simulink model "MoveMove"  (R2018a)
settings: Solver=ode4  StartTime=0.0  StopTime=19  FixedStep=5e-4  RelTol=1e-2
PostLoadFcn:
  | helperSetUp
values from neighbouring files (symbols this model uses):
  bf = 12    [data_vehicle.m]    (also in matlab.mat; testMotionPlanner.mat)
  br = 14    [data_vehicle.m]    (also in matlab.mat; testMotionPlanner.mat)
  Cd = .3    (= 0.3)    [data_vehicle.m]    (also in matlab.mat; myVehicle.m = this.CD; testMotionPlanner.mat)
  Cf = 1.3    [data_vehicle.m]    (also in forwardPropagate.m = 19000; matlab.mat; myVehicle.m = this.CF; testMotionPlanner.mat)
  costmap = vehicleCostmap(combinedMap, 'CellSize', res)    [creatCostmap.m]    (also in creatMyCostMap.m = vehicleCostmap(combinedMap, 'CellSize', res,                ; myMotionPlanning.m = vehicleCostmap(costmapStruct.Costs,          'FreeThreshold')
  Cr = 1.3    [data_vehicle.m]    (also in forwardPropagate.m = 33000; matlab.mat; myVehicle.m = this.CR; testMotionPlanner.mat)
  df = 0.95    [data_vehicle.m]    (also in matlab.mat; testMotionPlanner.mat)
  dr = 1    [data_vehicle.m]    (also in matlab.mat; testMotionPlanner.mat)
  Ef = -0.1    [data_vehicle.m]    (also in matlab.mat; testMotionPlanner.mat)
  Er = -0.1    [data_vehicle.m]    (also in matlab.mat; testMotionPlanner.mat)
  fv = .02    (= 0.02)    [data_vehicle.m]    (also in matlab.mat; testMotionPlanner.mat)
  Fzf = m*g*lr/l    (= 9879.29185185)    [data_vehicle.m]    (also in matlab.mat; testMotionPlanner.mat)
  Fzr = m*g*lf/l    (= 5811.34814815)    [data_vehicle.m]    (also in matlab.mat; testMotionPlanner.mat)
  g = 9.80665    [data_vehicle.m]    (also in matlab.mat; myVehicle.m = this.G; testMotionPlanner.mat)
  gB = 2/3    (= 0.666666666667)    [data_vehicle.m]    (also in matlab.mat; testMotionPlanner.mat)
  gT = 0    [data_vehicle.m]    (also in matlab.mat; testMotionPlanner.mat)
  Jz = 2200    [data_vehicle.m]    (also in matlab.mat; testMotionPlanner.mat)
  lf = 1    [data_vehicle.m]    (also in forwardPropagate.m = 1.2; matlab.mat; myVehicle.m = this.LF; testMotionPlanner.mat)
  lr = l-lf    (= 1.7)    [data_vehicle.m]    (also in forwardPropagate.m = 1.6; matlab.mat; myVehicle.m = this.LR; testMotionPlanner.mat)
  m = 1600    [data_vehicle.m]    (also in forwardPropagate.m = 1575; matlab.mat; myVehicle.m = this.M; testMotionPlanner.mat)
  mu = 1    [data_vehicle.m]    (also in matlab.mat; myVehicle.m = this.MU; testMotionPlanner.mat)
  psi0 = 0    [data_vehicle.m]    (also in matlab.mat; testMotionPlanner.mat)
  psip0 = 0    [data_vehicle.m]    (also in matlab.mat; testMotionPlanner.mat)
  rho = 1.2    [data_vehicle.m]    (also in matlab.mat; myVehicle.m = 1.29; testMotionPlanner.mat)
  S = 2    [data_vehicle.m]    (also in matlab.mat; testMotionPlanner.mat)
  vx0 = 0    [data_vehicle.m]    (also in matlab.mat; testMotionPlanner.mat)
  vy0 = 0    [data_vehicle.m]    (also in matlab.mat; testMotionPlanner.mat)
  XG0 = 0    [data_vehicle.m]    (also in matlab.mat; testMotionPlanner.mat)
  YG0 = 0    [data_vehicle.m]    (also in matlab.mat; testMotionPlanner.mat)
undefined symbols (not defined in the file or in its folder): dt_save
settings Model: Creator=jdrjk  LastModifiedBy=jdrjk

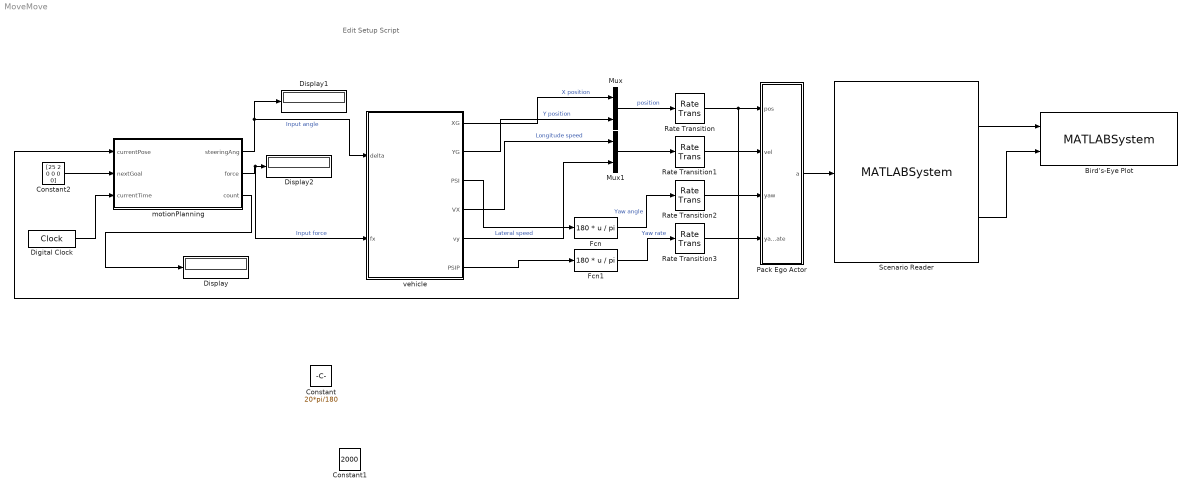
== system MoveMove ==
  note: Edit Setup Script
  Bird's-Eye Plot : MATLABSystem  System=helperBirdsEyePlot  ScenarioFileName=lkaScenarioSimulink  XLim=[-20, 50 ]  YLim=[ -30, 30 ]  HasActors=on  HasVision=off  HasRadar=off  HasTracks=off  TrackPositionSelector=[ 1, 0, 0, 0, 0, 0; 0, 0, 1, 0, 0, 0 ]  TrackVelocitySelector=[ 0, 1, 0, 0, 0, 0; 0, 0, 0, 1, 0, 0 ]  HasMIO=off  HasRoads=off  HasLaneBoundaries=off  HasLaneMarkings=on
      settings: ModelCloseFcn=helperCloseAll(gcb)
      mask Type: helperBirdsEyePlot
      mask Display:
      | disp(['Bird''s-Eye' char(10) 'Plot']);
      | port_label('input',1,'Actors');
      | port_label('input',2,'Lane Markings');
  Constant : Constant  Value=20*pi/180
  Constant1 : Constant  Value=2000
  Constant2 : Constant  Value=[25 2 0 0 0 0]  VectorParams1D=off
  Digital Clock : DigitalClock  SampleTime=0.01
  Display : Display
  Display1 : Display
  Display2 : Display
  Fcn : Fcn  Expr=180 * u / pi
  Fcn1 : Fcn  Expr=180 * u / pi
  Mux : Mux  Inputs=2
  Mux1 : Mux  Inputs=2
  Pack Ego Actor : MATLAB Function  TreatAsAtomicUnit=on
  Rate Transition{,1..3} (4 alike) : RateTransition  OutPortSampleTime=Ts
  Scenario Reader : MATLABSystem  System=helperScenarioReader  ScenarioFileName=lkaScenarioSimulink  EgoActorSource=Input port  EgoActorID=1  RoadBoundaries=off  LaneBoundaries=off  AllBoundaries=off  LaneBoundaryDistance=0:0.5:60  LaneBoundaryLocation=inner  CurrentLane=off  NumLanes=off  LaneMarkings=on  BusNameSource=Auto  BusName2Source=Auto  BusName3Source=Auto  SimulateUsing=Interpreted execution
      mask Type: helperScenarioReader
      mask Display:
      | disp(['Scenario' char(10) 'Reader']);
      | port_label('input',1,'Ego Actor');
      | port_label('output',1,'Actors');
      | port_label('output',2,'Lane Markings');
  motionPlanning : MATLAB Function  TreatAsAtomicUnit=on  mask{Costmap=costmap, MinIterations=1000, ConnectionDistance=3, MinTurningRadius=20, XStart=0, YStart=0, ThetaStart=0}
      mask prompts: Costmap "Vehicle costmap:"; MinIterations "Minimum iteration:"; ConnectionDistance "Connection distance [m]:"; MinTurningRadius "Minimum turning radius [m]:"; XStart "X positon [m]:"; YStart "Y position [m]:"; ThetaStart "Heading angle [deg]:"
      mask init:
      | validateattributes(Costmap, {'vehicleCostmap'}, {'scalar'});
      | 
      | startPose         = [XStart YStart ThetaStart 0 0 0];
      | varagout          = helperSLCreateUtilityStruct(Costmap);
      | vehicleDimsStruct = varagout{1};
      | costmapStruct     = varagout{2};
  vehicle : Subsystem
  wires:
  vehicle/4(VX) -> Mux1/1  "Longitude speed"
  vehicle/2(YG) -> Mux/2  "Y position"
  vehicle/5(vy) -> Mux1/2  "Lateral speed"
  vehicle/3(PSI) -> Fcn/1
  vehicle/1(XG) -> Mux/1  "X position"
  vehicle/6("PSIP ") -> Fcn1/1
  Rate Transition2/1 -> Pack Ego Actor/3(yaw)
  Mux1/1 -> Rate Transition1/1
  Rate Transition/1 -> motionPlanning/1(currentPose), Pack Ego Actor/1(pos)
  Scenario Reader/1 -> Bird's-Eye Plot/1
  Fcn1/1 -> Rate Transition3/1  "Yaw rate"
  Mux/1 -> Rate Transition/1  "position"
  Pack Ego Actor/1(a) -> Scenario Reader/1
  Rate Transition3/1 -> Pack Ego Actor/4(yawRate)
  Rate Transition1/1 -> Pack Ego Actor/2(vel)
  Fcn/1 -> Rate Transition2/1  "Yaw angle"
  Scenario Reader/2 -> Bird's-Eye Plot/2
  Constant2/1 -> motionPlanning/2(nextGoal)
  motionPlanning/2(force) -> vehicle/2(fx), Display2/1  "Input force"
  motionPlanning/3(count) -> Display/1
  Digital Clock/1 -> motionPlanning/3(currentTime)
  motionPlanning/1(steeringAng) -> vehicle/1(delta), Display1/1  "Input angle"

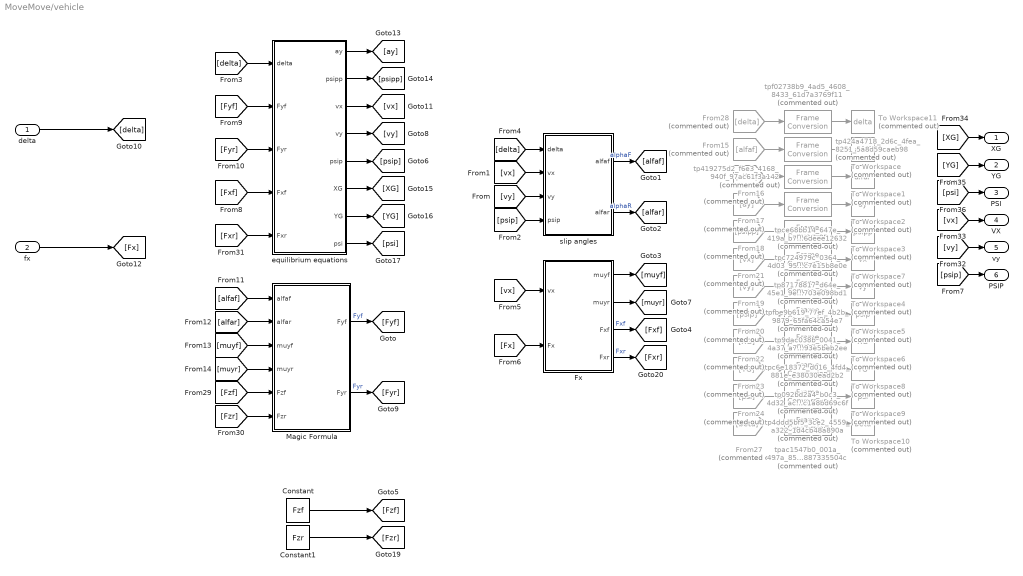
== system MoveMove/vehicle ==
  delta : Inport
  fx : Inport  Port=2
  Constant : Constant  Value=Fzf
  Constant1 : Constant  Value=Fzr
  From15 : From  Commented=on  GotoTag=alfaf
  From16 : From  Commented=on  GotoTag=alfar
  From17 : From  Commented=on  GotoTag=ay
  From18 : From  Commented=on  GotoTag=psipp
  From19 : From  Commented=on  GotoTag=vy
  From20 : From  Commented=on  GotoTag=psip
  From21 : From  Commented=on  GotoTag=vx
  From22 : From  Commented=on  GotoTag=XG
  From23 : From  Commented=on  GotoTag=YG
  From24 : From  Commented=on  GotoTag=psi
  From27 : From  Commented=on  GotoTag=beta
  From28 : From  Commented=on  GotoTag=delta
  Fx : Subsystem
  Magic Formula : Subsystem
  To Workspace : ToWorkspace  Commented=on  VariableName=alfaf  SampleTime=dt_save
  To Workspace1 : ToWorkspace  Commented=on  VariableName=alfar  SampleTime=dt_save
  To Workspace10 : ToWorkspace  Commented=on  VariableName=beta  SampleTime=dt_save
  To Workspace11 : ToWorkspace  Commented=on  VariableName=delta  SampleTime=dt_save
  To Workspace2 : ToWorkspace  Commented=on  VariableName=ay  SampleTime=dt_save
  To Workspace3 : ToWorkspace  Commented=on  VariableName=psipp  SampleTime=dt_save
  To Workspace4 : ToWorkspace  Commented=on  VariableName=vy  SampleTime=dt_save
  To Workspace5 : ToWorkspace  Commented=on  VariableName=psip  SampleTime=dt_save
  To Workspace6 : ToWorkspace  Commented=on  VariableName=XG  SampleTime=dt_save
  To Workspace7 : ToWorkspace  Commented=on  VariableName=vx  SampleTime=dt_save
  To Workspace8 : ToWorkspace  Commented=on  VariableName=YG  SampleTime=dt_save
  To Workspace9 : ToWorkspace  Commented=on  VariableName=psi  SampleTime=dt_save
  equilibrium equations : Subsystem
  slip angles : Subsystem
  tp092bd2a4_b0c3_4d32_ac59_7c1a8bd69c6f : FrameConversion  Commented=on  OutFrame=Sample-based
  tp419275d2_f6e3_4168_940f_97ac61f3a142 : FrameConversion  Commented=on  OutFrame=Sample-based
  tp424a4718_2d6c_4fea_8251_5a8d59caeb98 : FrameConversion  Commented=on  OutFrame=Sample-based
  tp4ddd5bf5_3ce2_4559_a322_1d4cb48a890a : FrameConversion  Commented=on  OutFrame=Sample-based
  tp87178817_d64e_45e1_9e30_db703e098bd1 : FrameConversion  Commented=on  OutFrame=Sample-based
  tp9dac038b_0041_4a37_a752_0593e5beb2ee : FrameConversion  Commented=on  OutFrame=Sample-based
  tpac1547b0_001a_497a_857c_68887335504c : FrameConversion  Commented=on  OutFrame=Sample-based
  tpc6e18372_d016_4fd4_881e_e38030ead2b2 : FrameConversion  Commented=on  OutFrame=Sample-based
  tpc724979c_0364_4d03_952a_37c7e15b8e0e : FrameConversion  Commented=on  OutFrame=Sample-based
  tpce68bb14_647e_419a_b744_5f6deee12632 : FrameConversion  Commented=on  OutFrame=Sample-based
  tpf02738b9_4ad5_4608_8433_61d7a3769f11 : FrameConversion  Commented=on  OutFrame=Sample-based
  tpfbe9b619_77ef_4b2b_9879_65fa64ca54e7 : FrameConversion  Commented=on  OutFrame=Sample-based
  XG : Outport
  YG : Outport  Port=2
  PSI : Outport  Port=3
  VX : Outport  Port=4
  vy : Outport  Port=5
  "PSIP " : Outport  Port=6
  wires:
  [psip] -> "PSIP "/1
  equilibrium equations/3(vx) -> [vx]
  [Fxr] -> equilibrium equations/5(Fxr)
  Constant/1 -> [Fzf]
  Constant1/1 -> [Fzr]
  From24/1 -> tp4ddd5bf5_3ce2_4559_a322_1d4cb48a890a/1
  tp9dac038b_0041_4a37_a752_0593e5beb2ee/1 -> To Workspace5/1
  From21/1 -> tp87178817_d64e_45e1_9e30_db703e098bd1/1
  From23/1 -> tp092bd2a4_b0c3_4d32_ac59_7c1a8bd69c6f/1
  From22/1 -> tpc6e18372_d016_4fd4_881e_e38030ead2b2/1
  tpfbe9b619_77ef_4b2b_9879_65fa64ca54e7/1 -> To Workspace4/1
  From19/1 -> tpfbe9b619_77ef_4b2b_9879_65fa64ca54e7/1
  tpc6e18372_d016_4fd4_881e_e38030ead2b2/1 -> To Workspace6/1
  tp87178817_d64e_45e1_9e30_db703e098bd1/1 -> To Workspace7/1
  From20/1 -> tp9dac038b_0041_4a37_a752_0593e5beb2ee/1
  tpc724979c_0364_4d03_952a_37c7e15b8e0e/1 -> To Workspace3/1
  tp4ddd5bf5_3ce2_4559_a322_1d4cb48a890a/1 -> To Workspace9/1
  tp092bd2a4_b0c3_4d32_ac59_7c1a8bd69c6f/1 -> To Workspace8/1
  tp419275d2_f6e3_4168_940f_97ac61f3a142/1 -> To Workspace1/1
  [Fzr] -> Magic Formula/6(Fzr)
  equilibrium equations/6(XG) -> [XG]
  equilibrium equations/1(ay) -> [ay]
  tpac1547b0_001a_497a_857c_68887335504c/1 -> To Workspace10/1
  equilibrium equations/7(YG) -> [YG]
  From27/1 -> tpac1547b0_001a_497a_857c_68887335504c/1
  tp424a4718_2d6c_4fea_8251_5a8d59caeb98/1 -> To Workspace/1
  [Fzf] -> Magic Formula/5(Fzf)
  equilibrium equations/2(psipp) -> [psipp]
  From18/1 -> tpc724979c_0364_4d03_952a_37c7e15b8e0e/1
  tpce68bb14_647e_419a_b744_5f6deee12632/1 -> To Workspace2/1
  From15/1 -> tp424a4718_2d6c_4fea_8251_5a8d59caeb98/1
  From16/1 -> tp419275d2_f6e3_4168_940f_97ac61f3a142/1
  fx/1 -> [Fx]
  equilibrium equations/8(psi) -> [psi]
  From17/1 -> tpce68bb14_647e_419a_b744_5f6deee12632/1
  tpf02738b9_4ad5_4608_8433_61d7a3769f11/1 -> To Workspace11/1
  From28/1 -> tpf02738b9_4ad5_4608_8433_61d7a3769f11/1
  Fx/3(Fxf) -> [Fxf]  "Fxf"
  Fx/2(muyr) -> [muyr]
  [delta] -> slip angles/1(delta)
  [alfaf] -> Magic Formula/1(alfaf)
  Fx/1(muyf) -> [muyf]
  delta/1 -> [delta]
  [vx] -> Fx/1(vx)
  [Fyr] -> equilibrium equations/3(Fyr)
  [psip] -> slip angles/4(psip)
  equilibrium equations/4(vy) -> [vy]
  [Fyf] -> equilibrium equations/2(Fyf)
  Magic Formula/1(Fyf) -> [Fyf]  "Fyf"
  slip angles/2(alfar) -> [alfar]  "alphaR"
  [muyr] -> Magic Formula/4(muyr)
  [vy] -> slip angles/3(vy)
  [muyf] -> Magic Formula/3(muyf)
  [alfar] -> Magic Formula/2(alfar)
  [Fxf] -> equilibrium equations/4(Fxf)
  Fx/4(Fxr) -> [Fxr]  "Fxr"
  [Fx] -> Fx/2(Fx)
  [vx] -> slip angles/2(vx)
  [delta] -> equilibrium equations/1(delta)
  equilibrium equations/5(psip) -> [psip]
  slip angles/1(alfaf) -> [alfaf]  "alphaF"
  Magic Formula/2(Fyr) -> [Fyr]  "Fyr"
  [vy] -> vy/1
  [YG] -> YG/1
  [XG] -> XG/1
  [psi] -> PSI/1
  [vx] -> VX/1

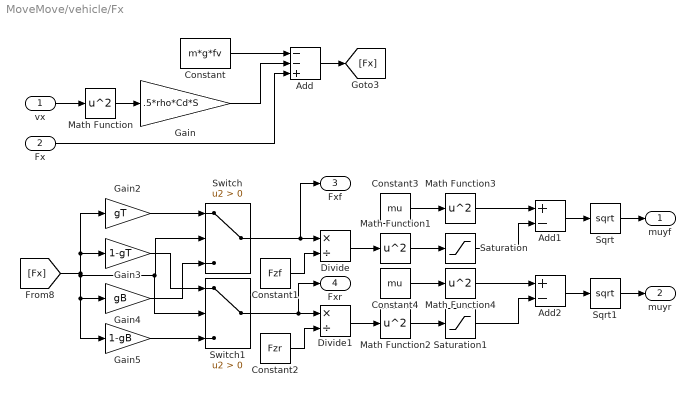
== system MoveMove/vehicle/Fx ==
  vx : Inport
  Fx : Inport  Port=2
  Add : Sum  Inputs=--+
  Add1 : Sum  Inputs=+-
  Add2 : Sum  Inputs=+-
  Constant : Constant  Value=m*g*fv
  Constant1 : Constant  Value=Fzf
  Constant2 : Constant  Value=Fzr
  Constant3 : Constant  Value=mu
  Constant4 : Constant  Value=mu
  Divide : Product  Inputs=*/
  Divide1 : Product  Inputs=*/
  Gain : Gain  Gain=.5*rho*Cd*S
  Gain2 : Gain  Gain=gT
  Gain3 : Gain  Gain=1-gT
  Gain4 : Gain  Gain=gB
  Gain5 : Gain  Gain=1-gB
  Math Function{,1..4} (5 alike) : Math  Operator=square  SaturateOnIntegerOverflow=on
  Saturation : Saturate  UpperLimit=1  LowerLimit=0
  Saturation1 : Saturate  UpperLimit=1  LowerLimit=0
  Sqrt : Sqrt  SaturateOnIntegerOverflow=on
  Sqrt1 : Sqrt  SaturateOnIntegerOverflow=on
  Switch : Switch  Criteria=u2 > Threshold
  Switch1 : Switch  Criteria=u2 > Threshold
  muyf : Outport
  muyr : Outport  Port=2
  Fxf : Outport  Port=3
  Fxr : Outport  Port=4
  wires:
  Math Function4/1 -> Add2/1
  Math Function3/1 -> Add1/1
  Sqrt/1 -> muyf/1
  Sqrt1/1 -> muyr/1
  Add2/1 -> Sqrt1/1
  Add1/1 -> Sqrt/1
  Saturation/1 -> Add1/2
  Saturation1/1 -> Add2/2
  Constant4/1 -> Math Function4/1
  Math Function2/1 -> Saturation1/1
  Math Function1/1 -> Saturation/1
  Divide1/1 -> Math Function2/1
  Divide/1 -> Math Function1/1
  Constant3/1 -> Math Function3/1
  Constant2/1 -> Divide1/2
  Constant1/1 -> Divide/2
  Switch1/1 -> Divide1/1, Fxr/1
  Switch/1 -> Divide/1, Fxf/1
  vx/1 -> Math Function/1
  Gain/1 -> Add/2
  Gain2/1 -> Switch/1
  Math Function/1 -> Gain/1
  Fx/1 -> Add/3
  Gain5/1 -> Switch1/3
  Gain3/1 -> Switch1/1
  [Fx] -> Gain4/1, Gain5/1, Switch/2, Switch1/2, Gain3/1, Gain2/1
  Add/1 -> [Fx]
  Gain4/1 -> Switch/3
  Constant/1 -> Add/1

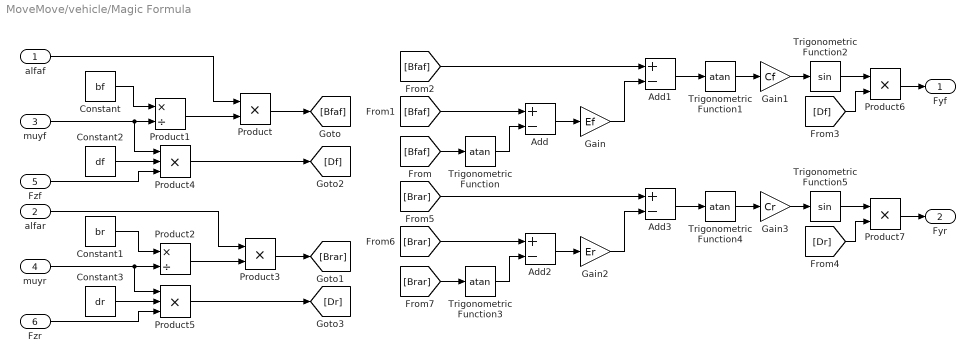
== system MoveMove/vehicle/Magic Formula ==
  alfaf : Inport
  alfar : Inport  Port=2
  muyf : Inport  Port=3
  muyr : Inport  Port=4
  Fzf : Inport  Port=5
  Fzr : Inport  Port=6
  Add{,1..3} (4 alike) : Sum  Inputs=+-
  Constant : Constant  Value=bf
  Constant1 : Constant  Value=br
  Constant2 : Constant  Value=df
  Constant3 : Constant  Value=dr
  Gain : Gain  Gain=Ef
  Gain1 : Gain  Gain=Cf
  Gain2 : Gain  Gain=Er
  Gain3 : Gain  Gain=Cr
  Product{,3,6..7} (4 alike) : Product
  Product1 : Product  Inputs=*/
  Product2 : Product  Inputs=*/
  Product4 : Product  Inputs=3
  Product5 : Product  Inputs=3
  Trigonometric Function{,1,3..4} (4 alike) : Trigonometry  Operator=atan
  Trigonometric Function2 : Trigonometry
  Trigonometric Function5 : Trigonometry
  Fyf : Outport
  Fyr : Outport  Port=2
  wires:
  Fzr/1 -> Product5/3
  Fzf/1 -> Product4/3
  Product7/1 -> Fyr/1
  [Brar] -> Trigonometric Function3/1
  Trigonometric Function3/1 -> Add2/2
  [Brar] -> Add2/1
  Add2/1 -> Gain2/1
  Gain2/1 -> Add3/2
  [Brar] -> Add3/1
  Add3/1 -> Trigonometric Function4/1
  Trigonometric Function4/1 -> Gain3/1
  Gain3/1 -> Trigonometric Function5/1
  Trigonometric Function5/1 -> Product7/1
  [Dr] -> Product7/2
  Product6/1 -> Fyf/1
  [Df] -> Product6/2
  Trigonometric Function2/1 -> Product6/1
  Gain1/1 -> Trigonometric Function2/1
  Trigonometric Function1/1 -> Gain1/1
  Add1/1 -> Trigonometric Function1/1
  [Bfaf] -> Add1/1
  Gain/1 -> Add1/2
  Add/1 -> Gain/1
  [Bfaf] -> Add/1
  Trigonometric Function/1 -> Add/2
  [Bfaf] -> Trigonometric Function/1
  Product5/1 -> [Dr]
  Product4/1 -> [Df]
  Constant3/1 -> Product5/2
  Constant2/1 -> Product4/2
  Product3/1 -> [Brar]
  Product/1 -> [Bfaf]
  alfar/1 -> Product3/1
  Product2/1 -> Product3/2
  alfaf/1 -> Product/1
  Product1/1 -> Product/2
  muyr/1 -> Product2/2, Product5/1
  Constant1/1 -> Product2/1
  muyf/1 -> Product1/2, Product4/1
  Constant/1 -> Product1/1

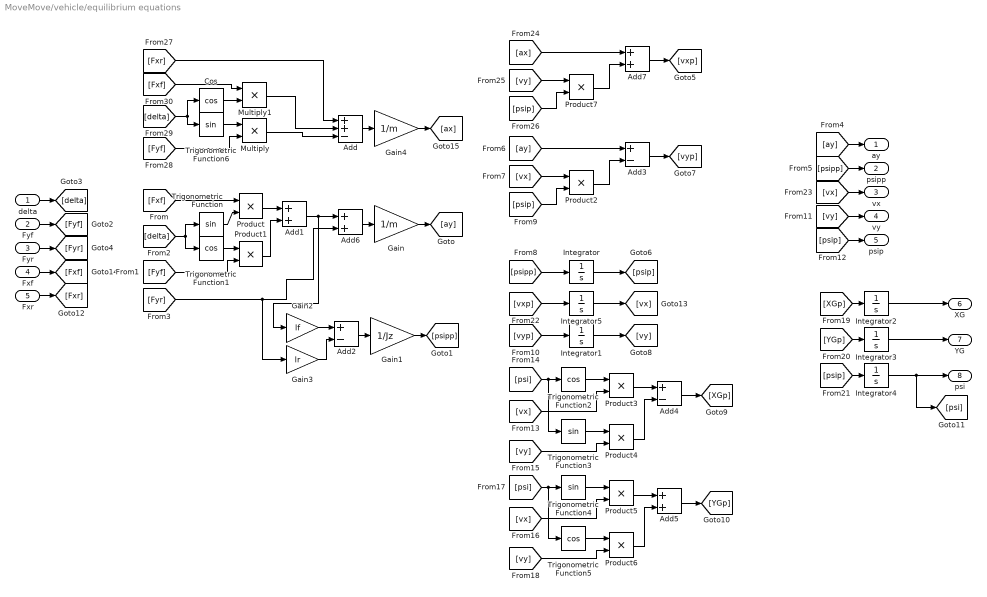
== system MoveMove/vehicle/equilibrium equations ==
  delta : Inport
  Fyf : Inport  Port=2
  Fyr : Inport  Port=3
  Fxf : Inport  Port=4
  Fxr : Inport  Port=5
  Add : Sum  Inputs=++-
  Add{1,5..7} (4 alike) : Sum
  Add2 : Sum  Inputs=+-
  Add3 : Sum  Inputs=+-
  Add4 : Sum  Inputs=+-
  Cos : Trigonometry  Operator=cos
  Gain : Gain  Gain=1/m
  Gain1 : Gain  Gain=1/Jz
  Gain2 : Gain  Gain=lf
  Gain3 : Gain  Gain=lr
  Gain4 : Gain  Gain=1/m
  Integrator : Integrator  InitialCondition=psip0  ContinuousStateAttributes='yaw_rate'
  Integrator1 : Integrator  InitialCondition=vy0  ContinuousStateAttributes='speed_y'
  Integrator2 : Integrator  InitialCondition=XG0  ContinuousStateAttributes='XG'
  Integrator3 : Integrator  InitialCondition=YG0  ContinuousStateAttributes='YG'
  Integrator4 : Integrator  InitialCondition=psi0  ContinuousStateAttributes='yaw'
  Integrator5 : Integrator  InitialCondition=vx0  ContinuousStateAttributes='yaw_rate'
  Multiply : Product
  Multiply1 : Product
  Product{,1..7} (8 alike) : Product
  Trigonometric Function{,3..4,6} (4 alike) : Trigonometry
  Trigonometric Function1 : Trigonometry  Operator=cos
  Trigonometric Function2 : Trigonometry  Operator=cos
  Trigonometric Function5 : Trigonometry  Operator=cos
  ay : Outport
  psipp : Outport  Port=2
  vx : Outport  Port=3
  vy : Outport  Port=4
  psip : Outport  Port=5
  XG : Outport  Port=6
  YG : Outport  Port=7
  psi : Outport  Port=8
  wires:
  Multiply1/1 -> Add/2
  Multiply/1 -> Add/3
  Cos/1 -> Multiply1/2
  [Fxf] -> Multiply1/1
  [Fyf] -> Multiply/2
  Trigonometric Function6/1 -> Multiply/1
  [delta] -> Cos/1, Trigonometric Function6/1
  [Fxr] -> Add/1
  Add/1 -> Gain4/1
  Gain4/1 -> [ax]
  Product7/1 -> Add7/2
  [psip] -> Product7/2
  [ax] -> Add7/1
  [vy] -> Product7/1
  Add7/1 -> [vxp]
  [vx] -> vx/1
  Integrator5/1 -> [vx]
  [vxp] -> Integrator5/1
  Fxr/1 -> [Fxr]
  Fxf/1 -> [Fxf]
  [psip] -> Integrator4/1
  Integrator4/1 -> psi/1, [psi]
  [YGp] -> Integrator3/1
  Integrator3/1 -> YG/1
  Integrator2/1 -> XG/1
  [XGp] -> Integrator2/1
  [psi] -> Trigonometric Function5/1, Trigonometric Function4/1
  Trigonometric Function4/1 -> Product5/1
  [vx] -> Product5/2
  Product5/1 -> Add5/1
  Trigonometric Function5/1 -> Product6/1
  [vy] -> Product6/2
  Product6/1 -> Add5/2
  Add5/1 -> [YGp]
  Add4/1 -> [XGp]
  Product4/1 -> Add4/2
  [vy] -> Product4/2
  Trigonometric Function3/1 -> Product4/1
  Product3/1 -> Add4/1
  [vx] -> Product3/2
  Trigonometric Function2/1 -> Product3/1
  [psi] -> Trigonometric Function2/1, Trigonometric Function3/1
  [psip] -> psip/1
  [vy] -> vy/1
  Integrator1/1 -> [vy]
  [vyp] -> Integrator1/1
  Add3/1 -> [vyp]
  Product2/1 -> Add3/2
  [ay] -> Add3/1
  [psip] -> Product2/2
  [vx] -> Product2/1
  Integrator/1 -> [psip]
  [psipp] -> Integrator/1
  [psipp] -> psipp/1
  Fyr/1 -> [Fyr]
  Gain2/1 -> Add2/1
  Gain3/1 -> Add2/2
  [Fyf] -> Product1/2
  Add2/1 -> Gain1/1
  Fyf/1 -> [Fyf]
  Add1/1 -> Add6/1, Gain2/1
  [Fxf] -> Product/1
  [ay] -> ay/1
  delta/1 -> [delta]
  Trigonometric Function1/1 -> Product1/1
  [delta] -> Trigonometric Function1/1, Trigonometric Function/1
  Gain/1 -> [ay]
  Product/1 -> Add1/1
  [Fyr] -> Gain3/1, Add6/2
  Gain1/1 -> [psipp]
  Add6/1 -> Gain/1
  Trigonometric Function/1 -> Product/2
  Product1/1 -> Add1/2

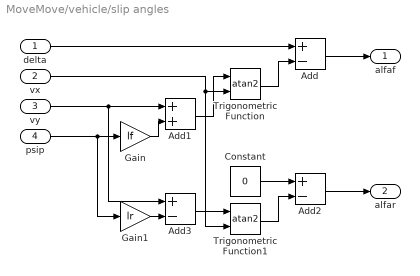
== system MoveMove/vehicle/slip angles ==
  delta : Inport
  vx : Inport  Port=2
  vy : Inport  Port=3
  psip : Inport  Port=4
  Add : Sum  Inputs=+-
  Add1 : Sum
  Add2 : Sum  Inputs=+-
  Add3 : Sum  Inputs=+-
  Constant : Constant  Value=0
  Gain : Gain  Gain=lf
  Gain1 : Gain  Gain=lr
  Trigonometric Function : Trigonometry  Operator=atan2
  Trigonometric Function1 : Trigonometry  Operator=atan2
  alfaf : Outport
  alfar : Outport  Port=2
  wires:
  Add2/1 -> alfar/1
  Add/1 -> alfaf/1
  delta/1 -> Add/1
  Trigonometric Function1/1 -> Add2/2
  Gain/1 -> Add1/2
  Add1/1 -> Trigonometric Function/1
  psip/1 -> Gain/1, Gain1/1
  vx/1 -> Trigonometric Function/2, Trigonometric Function1/2
  Gain1/1 -> Add3/2
  Trigonometric Function/1 -> Add/2
  Add3/1 -> Trigonometric Function1/1
  Constant/1 -> Add2/1
  vy/1 -> Add1/1, Add3/1

== matlab function MoveMove/motionPlanning ==
  data: steeringAng output double; force output double; currentPose input; nextGoal input; startPose parameter; costmapStruct parameter; vehicleDimsStruct parameter; ConnectionDistance parameter; MinTurningRadius parameter; MinIterations parameter; count output; currentTime input
function [steeringAng, force, count] = motionPlanning(currentPose, nextGoal, startPose, ...
    costmapStruct, vehicleDimsStruct, ...
    ConnectionDistance, MinTurningRadius, MinIterations, currentTime)

%motionPlanning plan a feasible path.

coder.extrinsic('myMotionPlanning');

controlOutput = zeros(1, 2);
controlOutput = myMotionPlanning(costmapStruct, vehicleDimsStruct, ...
    currentPose, nextGoal, startPose, ...
    MinIterations, ConnectionDistance, MinTurningRadius, currentTime);
steeringAng = controlOutput(1, 1);
force       = controlOutput(1, 2);

persistent counter;
if(isempty(counter))
    counter = 0;
end
counter = counter + 1;
count = counter;

== matlab function MoveMove/Pack Ego Actor ==
  data: pos input; a output Bus: BusActors1Actors size=1; vel input; yaw input; yawRate input
function a = packEgo(pos,vel,yaw,yawRate)
% Pack ego information into a single ego actor bus
%
% Imoprtant note:
% Output is a bus of type BusActorsActors. This is the same bus used by the
% helperScenarioReader to output an individual actor. If you change the
% output bus name of helperScenarioReader, change the output bus name here
% as well by clicking on 'Edit Data' in the menu above.

a = struct(...
    'ActorID',1,...
    'Position', [pos(1) pos(2) 0], ...
    'Velocity', [vel(1) vel(2) 0], ...
    'Roll', 0, ...
    'Pitch', 0, ...
    'Yaw', yaw, ...
    'AngularVelocity', [0 0 yawRate]);
